simulink model "approximator_test"  (R2016a)
settings: Solver=FixedStepAuto  StartTime=0.0  StopTime=30  FixedStep=0.01  MaxStep=0.001  RelTol=1e-3
undefined symbols (not defined in the file or in its folder): get, hot
libraries: tinbot x4, dspsnks4 x1
(part 2 of 2)

== stateflow chart approximator_test/Test Script ==
  state Start
    entry:
    motor_left = 2;
    motor_right = 2;
  state Step1
    entry:
    motor_left = 1;
    motor_right = -1;
  state Step2
    entry:
    motor_left = 2;
    motor_right = 2.5;
  state Step3
    entry:
    motor_left = 5;
    motor_right = 5;
  (default) -> Start
  Start -> Step1 : [after(5, sec)]
  Step1 -> Step2 : [after(5, sec)]
  Step2 -> Step3 : [after(5, sec)]
  data: motor_left output; motor_right output
